simulink model "Assignment3"  (R2022a)
settings: Solver=VariableStepAuto  StartTime=0.0  StopTime=70  RelTol=1e-3
settings Model: Creator=ahmed  LastModifiedBy=ahmed

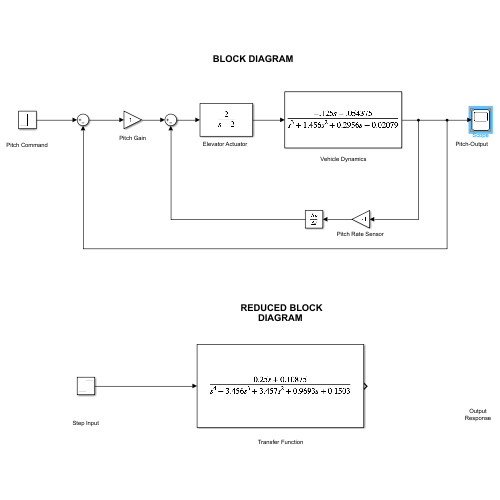
[thumbnail: Simulink's stored preview of the top-level diagram]
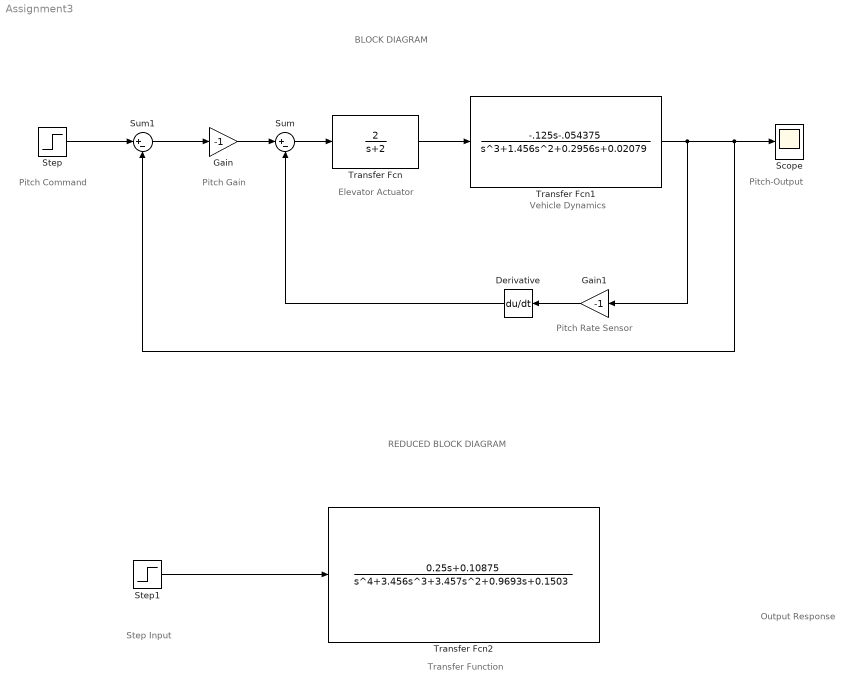
== system Assignment3 ==
  note: Transfer Function
  note: Output Response
  note: Step Input
  note: BLOCK DIAGRAM
  note: Pitch-Output
  note: Pitch Gain
  note: Vehicle Dynamics
  note: Elevator Actuator
  note: Pitch Command
  note: Pitch Rate Sensor
  note: REDUCED BLOCK DIAGRAM
  Derivative : Derivative
  Gain : Gain  Gain=-1
  Gain1 : Gain  Gain=-1
  Scope : Scope
  Step : Step  SampleTime=0
  Step1 : Step  SampleTime=0
  Sum : Sum  Inputs=|+-
  Sum1 : Sum  Inputs=|+-
  Transfer Fcn : TransferFcn  Numerator=[2]  Denominator=[1 2]
  Transfer Fcn1 : TransferFcn  Numerator=[-.125 -.054375]  Denominator=[1 1.456 0.2956 0.02079]
  Transfer Fcn2 : TransferFcn  Numerator=[0.25 0.10875]  Denominator=[1 3.456 3.457 0.9693 0.1503]
  wires:
  Gain/1 -> Sum/1
  Sum1/1 -> Gain/1
  Sum/1 -> Transfer Fcn/1
  Transfer Fcn/1 -> Transfer Fcn1/1
  Gain1/1 -> Derivative/1
  Transfer Fcn1/1 -> Gain1/1, Sum1/2, Scope/1
  Derivative/1 -> Sum/2
  Step/1 -> Sum1/1
  Step1/1 -> Transfer Fcn2/1
